simulink model "Copy_of_CM13_2024a_MachE_for_UA_HIL"  (R2024a)
settings: Solver=ode1  StartTime=0.0  StopTime=Inf  FixedStep=0.001  RelTol=1e-3  EnableMultiTasking=on
PreLoadFcn:
  | % if ~length(which('cmcmd')), cmenv; end
PostLoadFcn:
  | if any(exist('dsrtsu_mdlpostloadfcn', 'file') ~= 0), dsrtsu_mdlpostloadfcn('Execute', bdroot); end
InitFcn:
  | , if any(exist('rtifpga_mdlclblib', 'file') ~= 0), rtifpga_mdlclblib('Init', bdroot); end,
  | , if any(exist('dsmpb_private', 'file') ~= 0), dsmpb_private('dsmpb_mdlclblib', 'Init', bdroot); end,
undefined symbols (not defined in the file or in its folder): AccelCmd, ActTqLF_Nm_, ActTqLR_Nm_, ActTqRF_Nm_, ActTqRR_Nm_, BattChargeLimitMaxPwr, BattChargeLimitSocBpts, BattChargeLimitTbl, BattChrgCapcty, BattDischargeLimitSocBpts, BattDischargeLimitTbl, BattDischargeMaxPwr, BattNumCellsParallel, BattNumCellsSeries, BattOpenVoltCapBpts, BattOpenVoltTbl, BattResistSocBpts, BattResistTbl, BattResistTempBpts, BrakeMaxPrs, BrakeMaxTrq, ChassisDistCg2FrontAxle, ChassisDistCg2RearAxle, ChassisVehMass, CltchCmd, CoastDown, DecelCmd, DiffRatio, DiscIntNeverNeededParam, EnvGravCnst, EnvPrs, EnvTemp, FuelSpecificGrav, GearCmd, h, InitStates, lgSw, limitedMCT, MCT, MtrEffSpdBpts, MtrEffTbl, MtrEffTrqBpts, MtrPwrMax, MtrTrqMax, planned_speed, planned_time, pMCT, RealSimPara, ref_speed, Ref_speed, ref_time, Ref_time, rticanmm_blockfcn, rticanmm_initfcn, SteeringCmd, SupvsryCtrlRegenBrkCutOffTbl, SupvsryCtrlRegenSpdBpts, TestScnrioCycleNum, US06, VEH
libraries: simulink x264, VSIGenLib x262, etargetslib x201, dsmpblib x161, CarMaker4SL x142, rtimmsu_dsrtlib x32, vehdynlibtire x24, autolibshared x19, vehdynlibsuspension x14, vehdynlibtirecommon x14, autolibutils x10, VsrLibWheel x8
(part 34 of 47)

== system Copy_of_CM13_2024a_MachE_for_UA_HIL/Vehicle Under Test2/Vehicle/Vehicle Dynamics/Vehicle 14DOF/Wheels and Tires/VDBS/Tire2Veh ==
  Wheel : Inport
  Fz : Inport  Port=2
  WheelCamber : Inport  Port=3
  WheelSteer : Inport  Port=4
  Bus Creator : BusCreator  Inputs=2
  Bus Creator1 : BusCreator  Inputs=2
  Bus Selector7 : BusSelector  OutputSignals=Omega,Fx,Fy,Mz,Mx,My,Re,z,zdot,Kappa,Alpha
  Dead Zone2 : DeadZone  LowerValue=-5  UpperValue=5  ZeroCross=off
  Dead Zone3 : DeadZone  LowerValue=-10  UpperValue=10  ZeroCross=off
  Demux : Demux  Outputs=[2,2]
  Demux1 : Demux  Outputs=[2,2]
  Math Function : Math  Operator=transpose  SignedPower=on
  Reshape6 : Reshape  OutputDimensionality=Customize  OutputDimensions=[2,2]
  Routiong : Subsystem
  Vector Concatenate5 : Concatenate  Mode=Multidimensional array  ConcatenateDimension=2
  Vector Concatenate6 : Concatenate  Mode=Multidimensional array  ConcatenateDimension=2
  Vector Concatenate8 : Concatenate  NumInputs=3  Mode=Multidimensional array  ConcatenateDimension=2
  Wheel Angles : Subsystem
  Wheel to Body Transform : Subsystem
  Wheels : Outport  VectorParamsAs1DForOutWhenUnconnected=off
  Omega : Outport  Port=2  VectorParamsAs1DForOutWhenUnconnected=off
  FrntAxlF : Outport  Port=3  VectorParamsAs1DForOutWhenUnconnected=off
  RearAxlF : Outport  Port=4  VectorParamsAs1DForOutWhenUnconnected=off
  <Mz> : Outport  Port=5  VectorParamsAs1DForOutWhenUnconnected=off
  SuspWhlPz : Outport  Port=6  VectorParamsAs1DForOutWhenUnconnected=off
  SuspWhlVz : Outport  Port=7  VectorParamsAs1DForOutWhenUnconnected=off
  wires:
  Fz/1 -> Vector Concatenate8/3
  Vector Concatenate6/1 -> RearAxlF/1
  Vector Concatenate8/1 -> Math Function/1
  Demux/2 -> Vector Concatenate6/1
  Demux1/2 -> Vector Concatenate6/2
  Demux/1 -> Vector Concatenate5/1
  Math Function/1 -> Wheel to Body Transform/1(Forces)
  Dead Zone3/1 -> Vector Concatenate8/2
  Bus Selector7/2 -> Dead Zone2/1  "<Fx>"
  Dead Zone2/1 -> Vector Concatenate8/1
  Wheel to Body Transform/1(Fx) -> [Fx], Demux/1  "Fx"
  Vector Concatenate5/1 -> FrntAxlF/1
  Wheel/1 -> Bus Selector7/1
  Reshape6/1 -> Omega/1
  Demux1/1 -> Vector Concatenate5/2
  Wheel to Body Transform/2(Fy) -> Demux1/1, [Fy]  "Fy"
  Wheel Angles/1(Vehicle) -> Wheel to Body Transform/2(WheelAngles)
  Bus Selector7/1 -> [omega], Reshape6/1  "<Omega>"
  WheelSteer/1 -> Wheel Angles/1(Front), [WheelAngles]
  Bus Selector7/4 -> <Mz>/1, Routiong/1(<Mz>)  "<Mz>"
  Wheel to Body Transform/3(Fz) -> [Fz]
  WheelCamber/1 -> Wheel Angles/2(Camber), [CamberAngles]
  Bus Selector7/3 -> Dead Zone3/1  "<Fy>"
  Bus Selector7/5 -> Routiong/2(<Mx>)  "<Mx>"
  Bus Selector7/6 -> Routiong/3(<My>)  "<My>"
  Bus Selector7/7 -> Routiong/4(<Re>)  "<Re>"
  [omega] -> Routiong/9(Omega)  "omega"
  [Fx] -> Routiong/10(Fx)  "Fx"
  Bus Selector7/8 -> Routiong/5(<z>)  "<z>"
  [Fy] -> Routiong/11(Fy)  "Fy"
  [Fz] -> Routiong/12(Fz)  "Fz"
  Bus Selector7/9 -> Routiong/6(<zdot>)  "<zdot>"
  Bus Selector7/10 -> Routiong/7(<Kappa>)  "<Kappa>"
  Routiong/2(Out2) -> SuspWhlPz/1
  Routiong/3(Out3) -> SuspWhlVz/1
  [WheelAngles] -> Bus Creator/1  "Wheel Angles"
  Bus Creator1/1 -> Wheels/1  "Wheels"
  Routiong/1(Out1) -> Bus Creator1/1  "TireFrame"
  [CamberAngles] -> Bus Creator/2  "Camber Angles"
  Bus Creator/1 -> Bus Creator1/2  "Steering"
  Bus Selector7/11 -> Routiong/8(<Alpha>)  "<Alpha>"

== system Copy_of_CM13_2024a_MachE_for_UA_HIL/Vehicle Under Test2/Vehicle/Vehicle Dynamics/Vehicle 14DOF/Wheels and Tires/VDBS/Tires ==
  "DriveTorque " : Inport
  "Brake Pressure " : Inport  Port=2
  "r " : Inport  Port=3
  "Vx " : Inport  Port=4
  "Vy " : Inport  Port=5
  "Camber " : Inport  Port=6
  "Press " : Inport  Port=7
  "lambda " : Inport  Port=8
  "Gnd " : Inport  Port=9
  "FzSusp " : Inport  Port=10
  Fiala Tires : Subsystem  VariantControl=1
  MF Tires : Subsystem  VariantControl=0
  " Wheels" : Outport  VectorParamsAs1DForOutWhenUnconnected=off

== system Copy_of_CM13_2024a_MachE_for_UA_HIL/Vehicle Under Test2/Vehicle/Vehicle Dynamics/Vehicle 14DOF/Wheels and Tires/VDBS/Veh2Tire ==
  r : Inport
  Axle : Inport  Port=2
  Brake : Inport  Port=3
  VehVel : Inport  Port=4
  WheelSteer : Inport  Port=5
  WheelCamber : Inport  Port=6
  Demux4 : Demux
  Gain4 : Gain  Gain=[1;-1;1;-1]*0+1
  Mux1 : Mux
  Reshape3 : Reshape
  Reshape4 : Reshape
  Unary Minus : UnaryMinus
  Wheel Angles : Subsystem
  Wheel to Body Transform : Subsystem
  T : Outport  Unit=N*m  VectorParamsAs1DForOutWhenUnconnected=off
  P : Outport  Port=2  Unit=Pa  VectorParamsAs1DForOutWhenUnconnected=off
  psidot : Outport  Port=3  Unit=rad/s  VectorParamsAs1DForOutWhenUnconnected=off
  xdotAxle : Outport  Port=4  Unit=m/s  VectorParamsAs1DForOutWhenUnconnected=off
  ydotAxle : Outport  Port=5  Unit=m/s  VectorParamsAs1DForOutWhenUnconnected=off
  zdotAxle : Outport  Port=6  Unit=m/s  VectorParamsAs1DForOutWhenUnconnected=off
  wires:
  Demux4/1 -> Mux1/1
  Brake/1 -> Reshape3/1
  Demux4/4 -> Mux1/4
  Axle/1 -> Reshape4/1
  Wheel to Body Transform/1(xdotWheel) -> xdotAxle/1  "Vx"
  Demux4/2 -> Mux1/2
  Wheel to Body Transform/2(ydotWheel) -> ydotAxle/1  "Vy"
  WheelSteer/1 -> Wheel Angles/1(steer)
  Mux1/1 -> P/1
  r/1 -> Unary Minus/1
  Demux4/3 -> Mux1/3
  Reshape3/1 -> Demux4/1
  Gain4/1 -> T/1
  Reshape4/1 -> Gain4/1
  VehVel/1 -> Wheel to Body Transform/1(VelVeh)
  Wheel to Body Transform/3(zdotWheel) -> zdotAxle/1  "Vz"
  WheelCamber/1 -> Wheel Angles/2(camber)
  Unary Minus/1 -> psidot/1
  Wheel Angles/1(Vehicle) -> Wheel to Body Transform/2(WheelAngles)

== system Copy_of_CM13_2024a_MachE_for_UA_HIL/Vehicle Under Test2/Vehicle/Vehicle Dynamics/Vehicle 14DOF/Wheels and Tires/VDBS/scale factors with friction ==
  lamda_mu_x : Inport
  lamda_mu_y : Inport  Port=2
  0 : Constant  Value=[zeros(1,numWheels)]  VectorParams1D=off
  Reshape : Reshape  OutputDimensionality=Row vector (2-D)  OutputDimensions=[1,numWheels]
  Reshape1 : Reshape  OutputDimensionality=Row vector (2-D)  OutputDimensions=[1,numWheels]
  Signal Specification3 : SignalSpecification  Unit=1
  Vector Concatenate : Concatenate  NumInputs=5  Mode=Multidimensional array
  ones : Constant  Value=[ones(23,numWheels)]  VectorParams1D=off
  ones2 : Constant  Value=ones(1,numWheels)  VectorParams1D=off
  lambdas : Outport  Unit=1  VectorParamsAs1DForOutWhenUnconnected=off
  wires:
  lamda_mu_y/1 -> Reshape1/1
  lamda_mu_x/1 -> Reshape/1
  ones2/1 -> Vector Concatenate/1  "lambda_Fz0"
  Vector Concatenate/1 -> Signal Specification3/1
  ones/1 -> Vector Concatenate/5
  0/1 -> Vector Concatenate/4  "lamda_mu_V"
  Reshape1/1 -> Vector Concatenate/3
  Reshape/1 -> Vector Concatenate/2
  Signal Specification3/1 -> lambdas/1

== system Copy_of_CM13_2024a_MachE_for_UA_HIL/Vehicle Under Test2/Vehicle/Vehicle Dynamics/Vehicle 7DOF/Longitudinal Wheels 4DOF/Axle Forces/Bicycle ==
  F : Inport
  R : Inport  Port=2
  Sum of Elements : Sum  Inputs=+
  Sum of Elements1 : Sum  Inputs=+
  FrntAxlF : Outport  Unit=N  VectorParamsAs1DForOutWhenUnconnected=off
  RearAxlF : Outport  Port=2  Unit=N  VectorParamsAs1DForOutWhenUnconnected=off
  wires:
  Sum of Elements/1 -> FrntAxlF/1
  Sum of Elements1/1 -> RearAxlF/1
  R/1 -> Sum of Elements1/1
  F/1 -> Sum of Elements/1

== system Copy_of_CM13_2024a_MachE_for_UA_HIL/Vehicle Under Test2/Vehicle/Vehicle Dynamics/Vehicle 7DOF/Longitudinal Wheels 4DOF/Axle Forces/Dual ==
  F : Inport
  R : Inport  Port=2
  FrntAxlF : Outport  Unit=N  VectorParamsAs1DForOutWhenUnconnected=off
  RearAxlF : Outport  Port=2  Unit=N  VectorParamsAs1DForOutWhenUnconnected=off
  wires:
  R/1 -> RearAxlF/1
  F/1 -> FrntAxlF/1

== system Copy_of_CM13_2024a_MachE_for_UA_HIL/Vehicle Under Test2/Vehicle/Vehicle Dynamics/Vehicle 7DOF/Longitudinal Wheels 4DOF/Tires/4-by-1 Gnd ==
  Constant : Constant  Value=0
  Vector Concatenate : Concatenate  NumInputs=4
  Gnd : Outport
  wires:
  Constant/1 -> Vector Concatenate/4, Vector Concatenate/3, Vector Concatenate/2, Vector Concatenate/1
  Vector Concatenate/1 -> Gnd/1

== system Copy_of_CM13_2024a_MachE_for_UA_HIL/Vehicle Under Test2/Vehicle/Vehicle Dynamics/Vehicle 7DOF/Longitudinal Wheels 4DOF/Tires/4-by-1 Gnd1 ==
  Constant : Constant  Value=0
  Vector Concatenate : Concatenate  NumInputs=4
  Gnd : Outport
  wires:
  Constant/1 -> Vector Concatenate/4, Vector Concatenate/3, Vector Concatenate/2, Vector Concatenate/1
  Vector Concatenate/1 -> Gnd/1

== system Copy_of_CM13_2024a_MachE_for_UA_HIL/Vehicle Under Test2/Vehicle/Vehicle Dynamics/Vehicle 7DOF/Longitudinal Wheels 4DOF/Tires/4-by-1 Gnd2 ==
  Constant : Constant  Value=0
  Vector Concatenate : Concatenate  NumInputs=4
  Gnd : Outport
  wires:
  Constant/1 -> Vector Concatenate/4, Vector Concatenate/3, Vector Concatenate/2, Vector Concatenate/1
  Vector Concatenate/1 -> Gnd/1

== system Copy_of_CM13_2024a_MachE_for_UA_HIL/Vehicle Under Test2/Vehicle/Vehicle Dynamics/Vehicle 7DOF/Longitudinal Wheels 4DOF/Tires/4-by-1 Gnd3 ==
  Constant : Constant  Value=0
  Vector Concatenate : Concatenate  NumInputs=4
  Gnd : Outport
  wires:
  Constant/1 -> Vector Concatenate/4, Vector Concatenate/3, Vector Concatenate/2, Vector Concatenate/1
  Vector Concatenate/1 -> Gnd/1
